simulink model "pump_original"  (R2018a)
settings: Solver=VariableStepAuto  StartTime=0.0  StopTime=30  RelTol=1e-3
values from neighbouring files (symbols this model uses):
  Pl = 22    [pump_ori_perf.mat]
libraries: fl_lib x11, nesl_utility x6, sh_lib x4, simulink x3
settings Model: Creator=siwak  LastModifiedBy=siwak

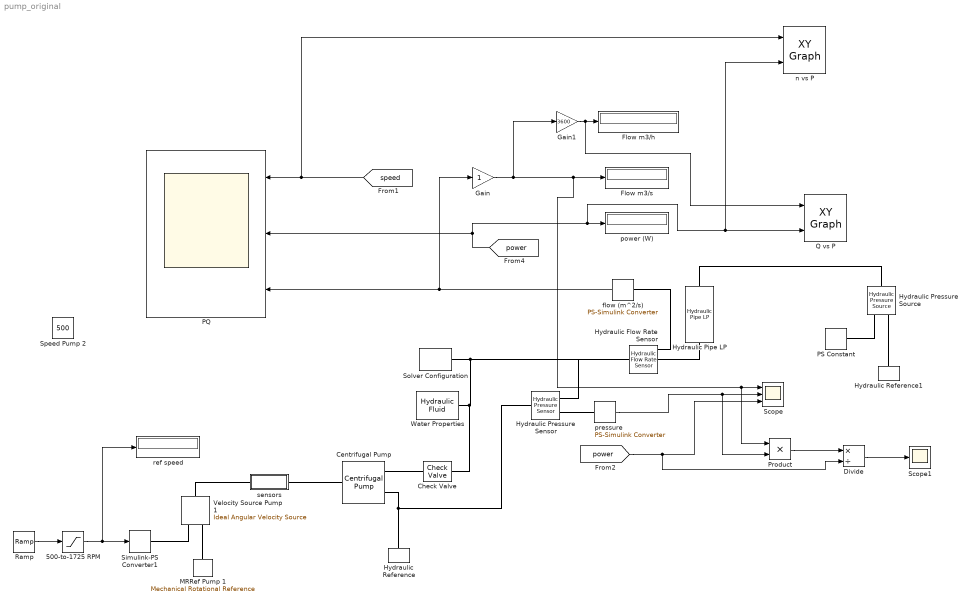
== system pump_original ==
  500-to-1725 RPM : Saturate  UpperLimit=1725  LowerLimit=500
  Centrifugal Pump : sh_lib/Pumps and Motors/Centrifugal Pump  mdl_type=2  c_1=326.8 Pa/(kg/m^3)  c_2=3.104e+4 Pa*s/kg  c_3=1.097e+7 Pa*s^2/(kg*m^3)  c_4=2.136e+5 Pa*s^2/(kg*m^3)  c_f=0.8  design_del=130 lpm  ref_velocity=1.77e+3 rpm  ref_density=940 kg/m^3  leak_resistance=1e+8 Pa/(m^3/s)  T_const=0.1 N*m  trq_press_coeff=1e-6 N*m/Pa  pump_del_1D="[0    0.0013    0.0041    0.0059    0.0069    0.0082] m^3/s"  press_diff_1D=[50.97 47.08 39.12 31.39 23.6 15.69] psi  pump_del_power_1D="[0    0.0013    0.0041    0.0059    0.0069    0.0082] m^3/s"  power_1D="[0    0.7800    2.1000    2.4000    2.1600    1.7000] HP"  pump_vel_2D=[ 3.2e+3 3.3e+3 3.4e+3 3.5e+3 ] rpm  pump_del_2D=[ 0 50 100 150 200 250 300 350 ] lpm  press_diff_2D=[ 8.3 8.8 9.3 9.9; 7.8 8.3 8.8 9.4; 7.2 7.6 8.2 8.7; 6.5 7 7.5 8; 5.6 6.1 6.6 7.1; 4.7 5.2 5.7 6.2; 3.4 4 4.4 4.9; 2.3 2.7 3.4 3.6 ] bar  pump_del_power_2D=[ 0 50 100 150 200 250 300 350 ] lpm  power_2D=[ 1.223e+3 1.341e+3 1.467e+3 1.6e+3; 1.414e+3 1.551e+3 1.696e+3 1.85e+3; 1.636e+3 1.794e+3 1.962e+3 2.14e+3; 1.941e+3 2.129e+3 2.326e+3 2.54e+3; 2.224e+3 2.439e+3 2.66e+3 2.91e+3; 2.453e+3 2.691e+3 2.947e+3 3.21e+3; 2.757e+3 3.024e+3 3.307e+3 3.608e+3; 2.945e+3 3.23e+3 3.533e+3 3.854e+3 ] W  omega_threshold=1e-9 rad/s  interp_method=1  extrap_method=1
      settings: SourceProductName=Simscape Fluids  SourceProductBaseCode=SH
  Check Valve : sh_lib/Valves/Directional Valves/Check Valve  area_max=506.7074790975 mm^2  pres_crack=0.01 psi  pres_max=0.1 psi  C_d=0.7  A_leak=1e-9 m^2  lam_spec=1  B_lam=0.999  Re_cr=12  dynamic=0  tau=0.1 s  area_init=1e-12 m^2
      settings: SourceProductName=Simscape Fluids  SourceProductBaseCode=SH
  Divide : Product  Inputs=*/
  Flow m3/h : Display
      settings: Decimation=2
  Flow m3/s : Display
      settings: Decimation=2
  Gain : Gain
  Gain1 : Gain  Gain=3600
  Hydraulic Flow Rate Sensor : fl_lib/Hydraulic/Hydraulic Sensors/Hydraulic Flow Rate Sensor
      settings: SourceProductName=Simscape
  Hydraulic Pipe LP : sh_lib/Low-Pressure Blocks/Hydraulic Pipe LP  cs_type=1  d_in=1 in  area=1e-4 m^2  D_h=1.12e-2 m  s_factor=64  length=Pl m  length_ad=1 m  roughness=15e-6 m  Re_lam=2000  Re_turb=4000  elevation_A=-0.5 m  elevation_B=Pl-0.5 m  g=9.80665 m/s^2  wall_type=1  pr_r_coef=2e-12 m/Pa  time_const=0.01 s  k_sh=1.4  p0=0 Pa
      settings: SourceProductName=Simscape Fluids  SourceProductBaseCode=SH
  Hydraulic Pressure Sensor : fl_lib/Hydraulic/Hydraulic Sensors/Hydraulic Pressure Sensor
      settings: SourceProductName=Simscape
  Hydraulic Pressure Source : fl_lib/Hydraulic/Hydraulic Sources/Hydraulic Pressure Source
      settings: SourceProductName=Simscape  SourceProductBaseCode=SS
  Hydraulic Reference : fl_lib/Hydraulic/Hydraulic Elements/Hydraulic Reference
      settings: SourceProductName=Simscape
  Hydraulic Reference1 : fl_lib/Hydraulic/Hydraulic Elements/Hydraulic Reference
      settings: SourceProductName=Simscape
  MRRef Pump 1 : fl_lib/Mechanical/Rotational Elements/Mechanical Rotational Reference
  PQ : Scope  NumInputPorts=3
  PS Constant : fl_lib/Physical Signals/Sources/PS Constant  constant=Pl/2
  Product : Product
  Q vs P : simulink/Sinks/XY Graph  xmin=0  xmax=11  ymin=0  ymax=8000  st=-1
  Ramp : simulink/Sources/Ramp  slope=60  start=0.1  InitialOutput=500
  Scope : Scope  NumInputPorts=3
  Scope1 : Scope
  Simulink-PS Converter1 : nesl_utility/Simulink-PS Converter  PhysicalDomain=network_engine_domain  SubClassName=ps_input  LeftPortType=input  RightPortType=output  PseudoPeriodic=off  Frequencies=[]  NoiseDistribution=none  NoiseParameters=[]  Unit=rpm  AffineConversion=off  FilteringAndDerivatives=zero  SimscapeFilterOrder=1  InputFilterTimeConstant=.001  UdotUserProvided=0
  Solver Configuration : nesl_utility/Solver Configuration  PhysicalDomain=network_engine_domain  SubClassName=solver  LeftPortType=input  RightPortType=generic  Tones=[]  Harmonics=[]  SimulateNoise=off  Profile=off  UseLocalSampling=off  EnableSwitchedLinearOptims=on  FrequencyDomain=off  UseCCode=off  RelTol=0.001  AbsTol=1e-06  MinStep=1e-09  ToWorkspace=off  RevertToSquareIcSolve=off  NumHomotopyIterations=100  PhasorMode=off  PhasorModeNumHarmonics=1  DoDC=off  ResidualTolerance=1e-9  UseLocalSolver=off  LocalSolverChoice=NE_BACKWARD_EULER_ADVANCER  LocalSolverSampleTime=.0001  DoFixedCost=off  MaxNonlinIter=3  MaxModeIter=2  LinearAlgebra=Sparse  EquationFormulation=NE_TIME_EF  DelaysMemoryBudget=1024  AutomaticFiltering=on  FilteringTimeConstant=0.001
  Speed Pump 2 : Constant  Value=500
  Velocity Source Pump 1 : fl_lib/Mechanical/Mechanical Sources/Ideal Angular Velocity Source
  Water Properties : sh_lib/Hydraulic Utilities/Hydraulic Fluid  DataSource=1  SelFluid=24  SysTemp=1  TrapAir=0.001  ViscDerFactor=1  range_error=2
      settings: SourceProductName=Simscape Fluids
  flow (m^2/s) : nesl_utility/PS-Simulink Converter  PhysicalDomain=network_engine_domain  SubClassName=ps_output  LeftPortType=input  RightPortType=output  PseudoPeriodic=off  Frequencies=[]  Unit=m^3/s  AffineConversion=off
  n vs P : simulink/Sinks/XY Graph  xmin=80  xmax=200  ymin=0  ymax=8000  st=-1
  power (W) : Display
      settings: Decimation=2
  pressure : nesl_utility/PS-Simulink Converter  PhysicalDomain=network_engine_domain  SubClassName=ps_output  LeftPortType=input  RightPortType=output  PseudoPeriodic=off  Frequencies=[]  Unit=Pa  AffineConversion=off
  ref speed : Display
      settings: Decimation=2
  sensors : Subsystem
  wires:
  flow (m^2/s)/1 -> Gain/1, PQ/3
  [power] -> PQ/2, n vs P/2, Q vs P/2, power (W)/1
  Gain1/1 -> Q vs P/1, Flow m3/h/1
  Ramp/1 -> 500-to-1725 RPM/1
  500-to-1725 RPM/1 -> ref speed/1, Simulink-PS Converter1/1
  [speed] -> n vs P/1, PQ/1
  pressure/1 -> Product/2, Scope/2
  [power] -> Divide/2, Scope/3
  Product/1 -> Divide/1
  Gain/1 -> Product/1, Scope/1, Flow m3/s/1, Gain1/1
  Divide/1 -> Scope1/1
  connections:
  Simulink-PS Converter1/RConn1 -- Velocity Source Pump 1/RConn1
  MRRef Pump 1/LConn1 -- Velocity Source Pump 1/RConn2
  Hydraulic Reference/LConn1 -- Hydraulic Pressure Sensor/LConn1 -- Centrifugal Pump/RConn2
  Hydraulic Pipe LP/LConn1 -- Hydraulic Flow Rate Sensor/RConn2
  Hydraulic Flow Rate Sensor/RConn1 -- flow (m^2/s)/LConn1
  Solver Configuration/RConn1 -- Hydraulic Pressure Sensor/RConn1 -- Hydraulic Flow Rate Sensor/LConn1 -- Check Valve/RConn1 -- Water Properties/RConn1
  Centrifugal Pump/RConn1 -- Check Valve/LConn1
  sensors/RConn1 -- Centrifugal Pump/LConn1
  sensors/LConn1 -- Velocity Source Pump 1/LConn1
  pressure/LConn1 -- Hydraulic Pressure Sensor/RConn2
  Hydraulic Pipe LP/RConn1 -- Hydraulic Pressure Source/LConn1
  Hydraulic Reference1/LConn1 -- Hydraulic Pressure Source/RConn2
  PS Constant/RConn1 -- Hydraulic Pressure Source/RConn1

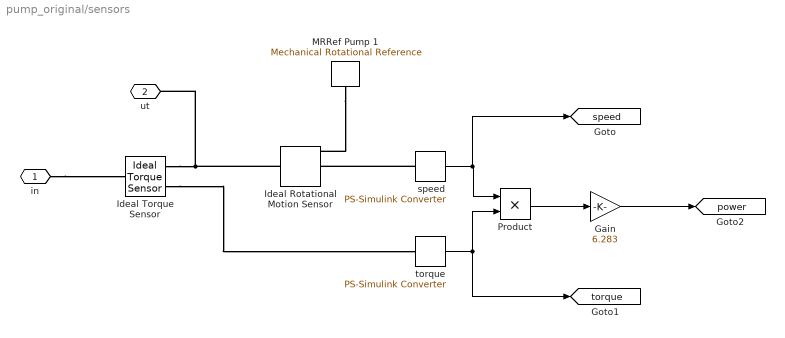
== system pump_original/sensors ==
  Gain : Gain  Gain=6.283
  Ideal Rotational Motion Sensor : fl_lib/Mechanical/Mechanical Sensors/Ideal Rotational Motion Sensor  offset=0 rad
  Ideal Torque Sensor : fl_lib/Mechanical/Mechanical Sensors/Ideal Torque Sensor
  MRRef Pump 1 : fl_lib/Mechanical/Rotational Elements/Mechanical Rotational Reference
  Product : Product
  speed : nesl_utility/PS-Simulink Converter  PhysicalDomain=network_engine_domain  SubClassName=ps_output  LeftPortType=input  RightPortType=output  PseudoPeriodic=off  Frequencies=[]  Unit=rad/s  AffineConversion=off
  torque : nesl_utility/PS-Simulink Converter  PhysicalDomain=network_engine_domain  SubClassName=ps_output  LeftPortType=input  RightPortType=output  PseudoPeriodic=off  Frequencies=[]  Unit=N*m  AffineConversion=off
  in : PMIOPort  Side=Left
  ut : PMIOPort  Port=2  Side=Right
  tag scope: power=global, speed=global, torque=global
  wires:
  speed/1 -> Product/1, [speed]
  torque/1 -> Product/2, [torque]
  Product/1 -> Gain/1
  Gain/1 -> [power]
  connections:
  in/RConn1 -- Ideal Torque Sensor/LConn1
  Ideal Torque Sensor/RConn1 -- Ideal Rotational Motion Sensor/LConn1 -- ut/RConn1
  MRRef Pump 1/LConn1 -- Ideal Rotational Motion Sensor/RConn1
  speed/LConn1 -- Ideal Rotational Motion Sensor/RConn2
  Ideal Torque Sensor/RConn2 -- torque/LConn1
